simulink model "forwardFlightModel"  (R2025a)
settings: Solver=VariableStepAuto  StartTime=0.0  StopTime=10.0  RelTol=1e-3
settings Model: Creator=Ayush_S  LastModifiedBy=Ayush_S

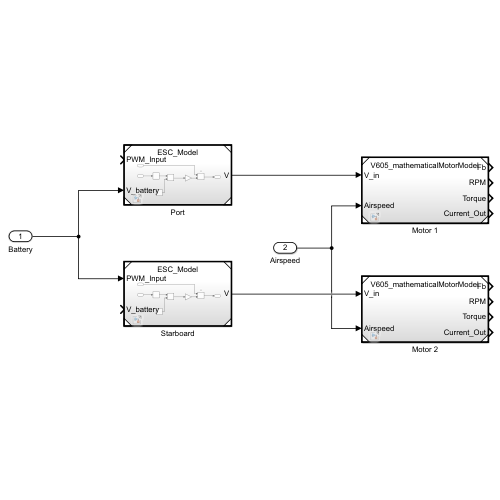
[thumbnail: Simulink's stored preview of the top-level diagram]
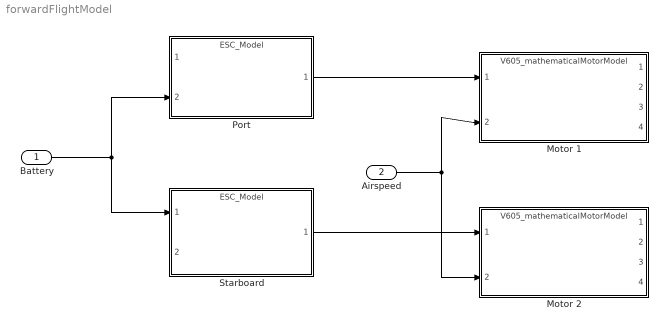
== system forwardFlightModel ==
  Battery : Inport
  Airspeed : Inport  Port=2
  Motor 1 : ModelReference  ModelNameDialog=V605_mathematicalMotorModel.slx  SimulationMode=Normal  ModelReferenceVersion=3.58
  Motor 2 : ModelReference  ModelNameDialog=V605_mathematicalMotorModel.slx  SimulationMode=Normal  ModelReferenceVersion=3.58
  Port : ModelReference  ModelNameDialog=ESC_Model.slx  SimulationMode=Normal  ModelReferenceVersion=1.9
  Starboard : ModelReference  ModelNameDialog=ESC_Model.slx  SimulationMode=Normal  ModelReferenceVersion=1.9
  wires:
  Port/1 -> Motor 1/1
  Starboard/1 -> Motor 2/1
  Airspeed/1 -> Motor 1/2, Motor 2/2
  Battery/1 -> Starboard/1, Port/2
